simulink model "toy_shape_threshold"  (R2020b)
settings: Solver=VariableStepAuto  StartTime=0.0  StopTime=100e-9  RelTol=1e-3
values from neighbouring files (symbols this model uses):
  v_threshold = (1.8/(2^9)) * 71    (= 0.249609375)    [zz_noShape.m]
libraries: simulink x1
settings Model: Creator=lydialee  LastModifiedBy=lydialee
settings SFSimCC: CustomCodeUndefinedFunction=UseInterfaceOnly

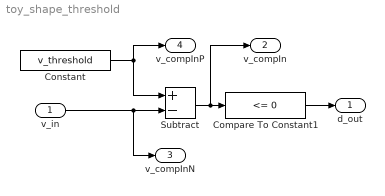
== system toy_shape_threshold ==
  v_in : Inport
  Compare To Constant1 : simulink/Logic and Bit Operations/Compare To Constant  relop=<=  const=0  OutDataTypeStr=uint8
  Constant : Constant  Value=v_threshold
  Subtract : Sum  Inputs=+-
  d_out : Outport  VectorParamsAs1DForOutWhenUnconnected=off
  v_compIn : Outport  Port=2  VectorParamsAs1DForOutWhenUnconnected=off
  v_compInN : Outport  Port=3  VectorParamsAs1DForOutWhenUnconnected=off
  v_compInP : Outport  Port=4  VectorParamsAs1DForOutWhenUnconnected=off
  wires:
  Compare To Constant1/1 -> d_out/1
  Subtract/1 -> v_compIn/1, Compare To Constant1/1
  Constant/1 -> v_compInP/1, Subtract/1
  v_in/1 -> v_compInN/1, Subtract/2
